simulink model "MicrogridControl"  (R2025b)
settings: Solver=VariableStepAuto  StartTime=0.0  StopTime=8  FixedStep=Ts  RelTol=1e-3
PreLoadFcn:
  | NormalOperation;
  | MicrogridControlParam;
undefined symbols (not defined in the file): base, bessModeInitial, bessSystem, bessVoltage, breakerStatus, DiscIntNeverNeededParam, ee_sli_rtmsupport, event, gcbh, generator, gflInverter, gfmInverter, Inertia, lineInductance, lineResistance, machine, plannedIsland, pmsm, powerLimit, powerQuality, PV, PVInverter, ref, resync, solar, solarInsolationChange, systemFrequency, Ts, windController, windSystem, windTurbine
libraries: nesl_utility x234, ee_lib x174, fl_lib x143, eeGeneralControl x137, simulink x78, eeTransforms x47, slpidlib x23, nesl_utility_internal x12, eePwmGenerator x9, eeSinusoidalMeasurementV2 x9, custom_lib x7, batteryecm_lib x6
(part 22 of 25)

== system MicrogridControl/Wind Farm/Wind Plant Integrated1/Detailed/Wind Turbine and Converters/Wind Plant/Back-to-Back Converters/Switching/Grid Side Converter ==
  mabc : Inport
  Add : Sum
  Constant1 : Constant
  Converter : ee_lib/Semiconductors & Converters/Converters/Converter (Three-Phase)  port_option=ee.enum.threePhasePort.composite  fidelity_option=ee.enum.converters.fidelity.detailed  device_type=ee.enum.converters.switchingdevice.ideal  showThermalPort=false  K=0  Vth=1 V  Vgt=1 V  Vgt_off=-1 V  Ih=1 A  Vf=0.8 V  Ron=0.001 Ohm  Rds=0.001 Ohm  Goff=1e-6 1/Ohm  Eon_scalar=22.86e-3 J  Eoff_scalar=17.14e-3 J  Eoff_natural_commutation=10e-3 J  Voff=300 V  Iout_scalar=600 A  onCurrentMeasDelay=0 s  useCurrentFromPreviousCycle=false  useVoltageFromPreviousCycle=false  diode_param=ee.enum.converters.protectiondiode.nodynamics  diode_Vf=0.01 V  diode_Ron=0.0001 Ohm  diode_Goff=1e-5 1/Ohm  diode_C=50 nF  diode_iRM=-235 A  diode_iF=300 A  diode_idot=-50 A/us  diode_trr_param=ee.enum.converters.diodetrr.trr_factor  diode_trr_factor=3  diode_trr=15 us  diode_Qrr=1500 s*uA  diode_rec_loss_model=ee.enum.diode.reverseRecoveryModel.fixed  diode_ErecVal=0 J  diode_scaleWithIandV=false  diode_ErecMat=zeros(2, 3) J  diode_TjrecVec=[298.15, 398.15] K  diode_IfrecVec=[.1, 1, 10] A  diode_IrecVal=10 A  diode_VrecVal=10 V  diode_tFilter=1 / 1000 / 100 s  thermal_network_parameterization=ee.enum.thermalNetworkTopology.external  Rth=[.08, .5] K/W  Rth_Cauer=[.08, .1, .5] K/W  Rth_Foster=[.08, .14, .22, .16] K/W  thermal_mass_parameterization=ee.enum.thermalNetwork.timeconstant  thermal_mass=[.01, .5] J/K  thermal_mass_Cauer=[.01, .1, .5] J/K  thermal_mass_Foster=[.001, .005, .05, .5] J/K  thermal_time_constant=[.001, .2] s  thermal_time_constant_Cauer=[.001, .1, .2] s  thermal_time_constant_Foster=[7e-05, .0007, .01, .08] s  thermal_mass_initial_temperatures=[25, 25] degC  thermal_mass_initial_temperatures_Cauer=[25, 25, 25] degC  junction_thermal_mass=0.01 J/K  Tvec_initial_Foster=[25, 25, 25, 25] degC  snubber_type=ee.enum.converters.snubber.exclude  Cs=1e-7 F  Rs=0.1 Ohm  Vce_loss=[0, 150, 300] V
  Demux : Demux  Outputs=3
  Demux1 : Demux  Outputs=3
  Gain : Gain  Gain=5
  Gain1 : Gain  Gain=0.5
  PWM Generator : eePwmGenerator/PWM Generator  CarrCount=Up  Tper=1/(fSw*1000)  Tdelay=0  Ts=1/(10*fSw*1000)
  Pulse Generation1 : Subsystem
  Rate Transition1 : RateTransition  OutPortSampleTime=1/(10*fSw*1000)
  Simulink-PS Converter{1..6} (6 alike) : nesl_utility/Simulink-PS Converter  PhysicalDomain=network_engine_domain  SubClassName=ps_input  LeftPortType=input  RightPortType=output  PseudoPeriodic=off  Frequencies=[]  NoiseDistribution=none  NoiseParameters=[]  Unit=1  AffineConversion=off  FilteringAndDerivatives=provide  SimscapeFilterOrder=1  InputFilterTimeConstant=0.001  UdotUserProvided=0
  Six-Pulse Gate Multiplexer : ee_lib/Semiconductors & Converters/Converters/Six-Pulse Gate Multiplexer  port_option=ee.enum.controlport.ps
  + : PMIOPort  Side=Left
  - : PMIOPort  Port=2  Side=Left
  ~ : PMIOPort  Port=3  Side=Right
  wires:
  [CH] -> Simulink-PS Converter2/1
  Demux/1 -> [AH]
  Add/1 -> Gain1/1
  Constant1/1 -> Add/2
  Demux/3 -> [CH]
  [AH] -> Simulink-PS Converter6/1
  Rate Transition1/1 -> PWM Generator/1
  [BH] -> Simulink-PS Converter4/1
  Demux1/3 -> [CL]
  [CL] -> Simulink-PS Converter1/1
  [AL] -> Simulink-PS Converter5/1
  PWM Generator/1 -> Gain/1
  Gain1/1 -> Rate Transition1/1
  Demux1/2 -> [BL]
  Demux/2 -> [BH]
  mabc/1 -> Add/1
  Gain/1 -> Pulse Generation1/1(G)
  Demux1/1 -> [AL]
  Pulse Generation1/2(G2) -> Demux1/1
  Pulse Generation1/1(G1) -> Demux/1
  [BL] -> Simulink-PS Converter3/1
  connections:
  +/RConn1 -- Converter/RConn1
  Six-Pulse Gate Multiplexer/LConn1 -- Simulink-PS Converter6/RConn1
  -/RConn1 -- Converter/RConn2
  Simulink-PS Converter2/RConn1 -- Six-Pulse Gate Multiplexer/LConn5
  Six-Pulse Gate Multiplexer/LConn3 -- Simulink-PS Converter4/RConn1
  Six-Pulse Gate Multiplexer/LConn2 -- Simulink-PS Converter5/RConn1
  Six-Pulse Gate Multiplexer/RConn1 -- Converter/LConn1
  ~/RConn1 -- Converter/LConn2
  Six-Pulse Gate Multiplexer/LConn4 -- Simulink-PS Converter3/RConn1
  Simulink-PS Converter1/RConn1 -- Six-Pulse Gate Multiplexer/LConn6

== system MicrogridControl/Wind Farm/Wind Plant Integrated1/Detailed/Wind Turbine and Converters/Wind Plant/Back-to-Back Converters/Switching/Machine Side Converter ==
  mabc : Inport
  Add : Sum
  Constant1 : Constant
  Converter : ee_lib/Semiconductors & Converters/Converters/Converter (Three-Phase)  port_option=ee.enum.threePhasePort.composite  fidelity_option=ee.enum.converters.fidelity.detailed  device_type=ee.enum.converters.switchingdevice.ideal  showThermalPort=false  K=0  Vth=1 V  Vgt=1 V  Vgt_off=-1 V  Ih=1 A  Vf=0.8 V  Ron=0.001 Ohm  Rds=0.001 Ohm  Goff=1e-6 1/Ohm  Eon_scalar=22.86e-3 J  Eoff_scalar=17.14e-3 J  Eoff_natural_commutation=10e-3 J  Voff=300 V  Iout_scalar=600 A  onCurrentMeasDelay=0 s  useCurrentFromPreviousCycle=false  useVoltageFromPreviousCycle=false  diode_param=ee.enum.converters.protectiondiode.nodynamics  diode_Vf=0.01 V  diode_Ron=0.0001 Ohm  diode_Goff=1e-5 1/Ohm  diode_C=50 nF  diode_iRM=-235 A  diode_iF=300 A  diode_idot=-50 A/us  diode_trr_param=ee.enum.converters.diodetrr.trr_factor  diode_trr_factor=3  diode_trr=15 us  diode_Qrr=1500 s*uA  diode_rec_loss_model=ee.enum.diode.reverseRecoveryModel.fixed  diode_ErecVal=0 J  diode_scaleWithIandV=false  diode_ErecMat=zeros(2, 3) J  diode_TjrecVec=[298.15, 398.15] K  diode_IfrecVec=[.1, 1, 10] A  diode_IrecVal=10 A  diode_VrecVal=10 V  diode_tFilter=1 / 1000 / 100 s  thermal_network_parameterization=ee.enum.thermalNetworkTopology.external  Rth=[.08, .5] K/W  Rth_Cauer=[.08, .1, .5] K/W  Rth_Foster=[.08, .14, .22, .16] K/W  thermal_mass_parameterization=ee.enum.thermalNetwork.timeconstant  thermal_mass=[.01, .5] J/K  thermal_mass_Cauer=[.01, .1, .5] J/K  thermal_mass_Foster=[.001, .005, .05, .5] J/K  thermal_time_constant=[.001, .2] s  thermal_time_constant_Cauer=[.001, .1, .2] s  thermal_time_constant_Foster=[7e-05, .0007, .01, .08] s  thermal_mass_initial_temperatures=[25, 25] degC  thermal_mass_initial_temperatures_Cauer=[25, 25, 25] degC  junction_thermal_mass=0.01 J/K  Tvec_initial_Foster=[25, 25, 25, 25] degC  snubber_type=ee.enum.converters.snubber.exclude  Cs=1e-7 F  Rs=0.1 Ohm  Vce_loss=[0, 150, 300] V
  Demux : Demux  Outputs=3
  Demux1 : Demux  Outputs=3
  Gain : Gain  Gain=5
  Gain1 : Gain  Gain=0.5
  PWM Generator : eePwmGenerator/PWM Generator  CarrCount=Up  Tper=1/(fSw*1000)  Tdelay=0  Ts=1/(10*fSw*1000)
  Pulse Generation : Subsystem
  Rate Transition1 : RateTransition  OutPortSampleTime=1/(10*fSw*1000)
  Simulink-PS Converter{1..6} (6 alike) : nesl_utility/Simulink-PS Converter  PhysicalDomain=network_engine_domain  SubClassName=ps_input  LeftPortType=input  RightPortType=output  PseudoPeriodic=off  Frequencies=[]  NoiseDistribution=none  NoiseParameters=[]  Unit=1  AffineConversion=off  FilteringAndDerivatives=provide  SimscapeFilterOrder=1  InputFilterTimeConstant=0.001  UdotUserProvided=0
  Six-Pulse Gate Multiplexer : ee_lib/Semiconductors & Converters/Converters/Six-Pulse Gate Multiplexer  port_option=ee.enum.controlport.ps
  + : PMIOPort  Side=Left
  - : PMIOPort  Port=2  Side=Left
  ~ : PMIOPort  Port=3  Side=Right
  wires:
  Demux1/1 -> [AL]
  Rate Transition1/1 -> PWM Generator/1
  Gain/1 -> Pulse Generation/1(G)
  [BH] -> Simulink-PS Converter4/1
  Gain1/1 -> Rate Transition1/1
  Demux/2 -> [BH]
  Pulse Generation/1(G1) -> Demux/1
  Pulse Generation/2(G2) -> Demux1/1
  PWM Generator/1 -> Gain/1
  Constant1/1 -> Add/2
  [AL] -> Simulink-PS Converter5/1
  Demux/3 -> [CH]
  [BL] -> Simulink-PS Converter3/1
  Demux/1 -> [AH]
  Add/1 -> Gain1/1
  Demux1/2 -> [BL]
  [CH] -> Simulink-PS Converter2/1
  Demux1/3 -> [CL]
  [CL] -> Simulink-PS Converter1/1
  mabc/1 -> Add/1
  [AH] -> Simulink-PS Converter6/1
  connections:
  Simulink-PS Converter2/RConn1 -- Six-Pulse Gate Multiplexer/LConn5
  ~/RConn1 -- Converter/LConn2
  Six-Pulse Gate Multiplexer/RConn1 -- Converter/LConn1
  Six-Pulse Gate Multiplexer/LConn2 -- Simulink-PS Converter5/RConn1
  Six-Pulse Gate Multiplexer/LConn4 -- Simulink-PS Converter3/RConn1
  -/RConn1 -- Converter/RConn2
  Six-Pulse Gate Multiplexer/LConn1 -- Simulink-PS Converter6/RConn1
  +/RConn1 -- Converter/RConn1
  Simulink-PS Converter1/RConn1 -- Six-Pulse Gate Multiplexer/LConn6
  Six-Pulse Gate Multiplexer/LConn3 -- Simulink-PS Converter4/RConn1

== system MicrogridControl/BESS/BESS Integrated/Detailed/BESS Controller/Grid Forming/Current Limiting/CurrentLimitingMethod/currentLimitAndVirtual/Current Saturation ==
  note: Vs-delV
  Id : Inport
  Iq : Inport  Port=2
  Imaxsat : Inport  Port=3
  Enable : EnablePort
  Compare : Subsystem
  Constant1 : Constant  Value=0
  Constant2 : Constant  Value=0
  If : If
  If Action Subsystem : Subsystem  TreatAsAtomicUnit=on
  If Action Subsystem1 : Subsystem  TreatAsAtomicUnit=on
  Math Function : Math  Operator=hypot
  Merge : Merge
  Merge1 : Merge
  Subtract : Sum  Inputs=+-
  delVd : Outport
  delVq : Outport  Port=2
  idmax : Outport  Port=3
  iqmax : Outport  Port=4
  wires:
  [Imax] -> If Action Subsystem/4(maxI)
  Imaxsat/1 -> Subtract/1, [Imax]
  Merge1/1 -> iqmax/1
  [Isq] -> If Action Subsystem/3(Isq)
  Constant1/1 -> delVd/1
  [Isd] -> If Action Subsystem/2(Isd)
  Merge/1 -> idmax/1
  If Action Subsystem1/2(Iqmax) -> Merge1/2
  Id/1 -> Math Function/1, [Isd]
  [Is] -> If Action Subsystem/1(Is)
  If Action Subsystem/1(Idmax) -> Merge/1
  Compare/1(Out1) -> If/1
  Subtract/1 -> Compare/1(u)
  If Action Subsystem/2(Iqmax) -> Merge1/1
  If/2 -> If Action Subsystem1/Action
  Math Function/1 -> Subtract/2, [Is]
  Constant2/1 -> delVq/1
  If Action Subsystem1/1(Idmax) -> Merge/2
  If/1 -> If Action Subsystem/Action
  Iq/1 -> Math Function/2, [Isq]

== system MicrogridControl/BESS/BESS Integrated/Detailed/BESS Controller/Grid Forming/Current Limiting/CurrentLimitingMethod/currentLimitAndVirtual/No Fault Ride Through ==
  Id : Inport
  Iq : Inport  Port=2
  Enable : EnablePort
  Constant{1..4} (4 alike) : Constant  Value=0
  Terminator : Terminator
  Terminator1 : Terminator
  delVd : Outport
  delVq : Outport  Port=2
  idmax : Outport  Port=3
  iqmax : Outport  Port=4
  wires:
  Iq/1 -> Terminator1/1
  Id/1 -> Terminator/1
  Constant4/1 -> delVq/1
  Constant1/1 -> delVd/1
  Constant2/1 -> idmax/1
  Constant3/1 -> iqmax/1

== system MicrogridControl/BESS/BESS Integrated/Detailed/BESS Controller/Grid Forming/Current Limiting/CurrentLimitingMethod/currentLimitAndVirtual/VI ==
  note: X/R ratio
  note: Resistance coefficient
  Id : Inport
  Iq : Inport  Port=2
  Imax : Inport  Port=3
  Enable : EnablePort
  Constant1 : Constant  Value=0
  Constant2 : Constant  Value=0
  Constant3 : Constant  Value=0
  Gain : Gain  Gain=ctLimitVirtualImp
  Gain1 : Gain  Gain=ctLimitXbyR
  Low-Pass Filter : eeGeneralControl/Low-Pass Filter (Discrete or Continuous)  K=1  T=currentVITimeConst  B=inf  A=-inf  init_option=Inherited from block input  x0=0  Ts=-1
  Math Function : Math  Operator=hypot
  Product{,1..3} (4 alike) : Product
  Relay1 : Relay  OnSwitchValue=0.01  OffSwitchValue=-0.1
  Saturation : Saturate  UpperLimit=1  LowerLimit=-1
  Saturation1 : Saturate  UpperLimit=1  LowerLimit=-1
  Sum : Sum  Inputs=|+-
  Sum1 : Sum  Inputs=|+-
  Sum2 : Sum  Inputs=++|
  Switch : Switch  Criteria=u2 > Threshold  SaturateOnIntegerOverflow=off  InputSameDT=off
  delVd : Outport
  delVq : Outport  Port=2
  idmax : Outport  Port=3
  iqmax : Outport  Port=4
  wires:
  Imax/1 -> Sum/2  "IsMaximum"
  Low-Pass Filter/1 -> Sum/1
  Relay1/1 -> Switch/2
  Constant2/1 -> idmax/1
  Constant3/1 -> iqmax/1
  Saturation/1 -> delVd/1
  Constant1/1 -> Switch/3
  Gain/1 -> Switch/1
  Product2/1 -> Sum1/2
  Product1/1 -> Sum2/1
  Saturation1/1 -> delVq/1
  [Igd] -> Product/2, Product1/1
  Switch/1 -> Gain1/1, Product/1, Product3/2
  Math Function/1 -> Low-Pass Filter/1  "Is"
  Iq/1 -> Math Function/2, [Igq]
  [Igq] -> Product2/2, Product3/1
  Product/1 -> Sum1/1
  Sum1/1 -> Saturation/1
  Sum/1 -> Relay1/1, Gain/1
  Sum2/1 -> Saturation1/1
  Id/1 -> [Igd], Math Function/1
  Product3/1 -> Sum2/2
  Gain1/1 -> Product2/1, Product1/2

== system MicrogridControl/BESS/BESS Integrated/Detailed/BESS Controller/Grid Forming/Current Limiting/CurrentLimitingMethod/currentSaturation/Compare ==
  u : Inport
  AND : Logic  IconShape=distinctive  AllPortsSameDT=off  OutDataTypeStr=boolean
  Compare To Constant : simulink/Logic and Bit Operations/Compare To Constant  relop=>  const=ctLimitDelayTime  OutDataTypeStr=boolean
  Compare To Zero : simulink/Logic and Bit Operations/Compare To Zero  relop=<=  OutDataTypeStr=boolean
  Data Type Conversion : DataTypeConversion  SaturateOnIntegerOverflow=off  RndMeth=Floor
  Data Type Conversion1 : DataTypeConversion  SaturateOnIntegerOverflow=off  RndMeth=Floor
  Discrete-Time Integrator : DiscreteIntegrator  IntegratorMethod=Integration: Backward Euler  ExternalReset=level  SampleTime=currentControlTs  LimitOutput=on  UpperSaturationLimit=ctLimitDelayTime*2  LowerSaturationLimit=0  ICPrevOutput=DiscIntNeverNeededParam  ICPrevScaledInput=DiscIntNeverNeededParam
  Out1 : Outport
  wires:
  Data Type Conversion1/1 -> AND/1, Discrete-Time Integrator/1, Discrete-Time Integrator/2
  Data Type Conversion/1 -> Out1/1
  Discrete-Time Integrator/1 -> Compare To Constant/1
  u/1 -> Compare To Zero/1
  Compare To Constant/1 -> AND/2
  Compare To Zero/1 -> Data Type Conversion1/1
  AND/1 -> Data Type Conversion/1

== system MicrogridControl/BESS/BESS Integrated/Detailed/BESS Controller/Grid Forming/Current Limiting/CurrentLimitingMethod/currentSaturation/If Action Subsystem ==
  Is : Inport
  Isd : Inport  Port=2
  Isq : Inport  Port=3
  Action Port : ActionPort  ActionPortLabel=if(u1 > 0)
  Constant : Constant  Value=maxSatCurrentLimit
  Divide : Product  Inputs=*/
  Product : Product
  Product1 : Product
  Idmax : Outport
  Iqmax : Outport  Port=2
  wires:
  Product/1 -> Iqmax/1
  Product1/1 -> Idmax/1
  Isq/1 -> Product/2
  Isd/1 -> Product1/1
  Divide/1 -> Product/1, Product1/2
  Is/1 -> Divide/2
  Constant/1 -> Divide/1

== system MicrogridControl/BESS/BESS Integrated/Detailed/BESS Controller/Grid Forming/Current Limiting/CurrentLimitingMethod/currentSaturation/If Action Subsystem1 ==
  Action Port : ActionPort  ActionPortLabel=else
  Constant3 : Constant  Value=0
  Constant4 : Constant  Value=0
  Idmax : Outport
  Iqmax : Outport  Port=2
  wires:
  Constant3/1 -> Idmax/1
  Constant4/1 -> Iqmax/1

== system MicrogridControl/BESS/BESS Integrated/Detailed/BESS Controller/Grid Forming/Grid Voltage Reactive Power Support/Modifying Reactive Power Reference/Changing the Power Reference/ActivePowerReference ==
  note: Ensure Pref sign is maintained
  Id : Inport
  Vd : Inport  Port=2
  Pref : Inport  Port=3
  Abs1 : Abs  SaturateOnIntegerOverflow=off
  Abs2 : Abs  SaturateOnIntegerOverflow=off
  Min : MinMax  Inputs=2
  Product : Product
  Product2 : Product
  Saturation : Saturate  UpperLimit=1  LowerLimit=-1
  Sign : Signum
  PrefNew : Outport
  wires:
  Saturation/1 -> PrefNew/1
  Vd/1 -> Product/2
  Abs2/1 -> Min/1
  Product2/1 -> Saturation/1
  Min/1 -> Product2/1
  Product/1 -> Abs2/1
  Abs1/1 -> Min/2
  Sign/1 -> Product2/2
  Id/1 -> Product/1
  Pref/1 -> Sign/1, Abs1/1

== system MicrogridControl/BESS/BESS Integrated/Detailed/BESS Controller/Grid Forming/Grid Voltage Reactive Power Support/Modifying Reactive Power Reference/Changing the Power Reference/EstimateIdForGivenIq ==
  Iq : Inport
  Add Constant1 : Bias  Bias=1*1  SaturateOnIntegerOverflow=off
  Gain : Gain  Gain=-1
  Gain3 : Gain  Gain=0.9
  Sqrt : Sqrt
  Square : Math  Operator=square
  Id : Outport
  wires:
  Iq/1 -> Square/1
  Add Constant1/1 -> Sqrt/1
  Sqrt/1 -> Gain3/1
  Gain/1 -> Add Constant1/1
  Gain3/1 -> Id/1
  Square/1 -> Gain/1

== system MicrogridControl/BESS/BESS Integrated/Detailed/BESS Controller/Grid Forming/Grid Voltage Reactive Power Support/Modifying Reactive Power Reference/Changing the Power Reference/EstimateIqForReactivePower ==
  note: Computing minimum reactive power as per GC0137
  Vmin : Inport
  Vd : Inport  Port=2
  Vs : Inport  Port=3
  Abs : Abs  SaturateOnIntegerOverflow=off
  Add : Sum
  Add Constant : Bias  Bias=1  SaturateOnIntegerOverflow=off
  GC0137 line slope : Gain  Gain=-1.4578
  Gain4 : Gain  Gain=1.5
  Saturation : Saturate  UpperLimit=1  LowerLimit=0
  Saturation1 : Saturate  UpperLimit=1  LowerLimit=-1
  Subtract : Sum  Inputs=+-
  Iq : Outport
  wires:
  Add Constant/1 -> Add/2
  Saturation/1 -> Iq/1
  Add/1 -> Saturation/1
  Vd/1 -> Subtract/2
  Vs/1 -> Abs/1
  Vmin/1 -> Subtract/1
  Gain4/1 -> Saturation1/1
  Saturation1/1 -> Add/1
  Subtract/1 -> Gain4/1
  GC0137 line slope/1 -> Add Constant/1
  Abs/1 -> GC0137 line slope/1

== system MicrogridControl/BESS/BESS Integrated/Detailed/BESS Controller/Grid Forming/Grid Voltage Reactive Power Support/Modifying Reactive Power Reference/Changing the Power Reference/ReactivePowerReference ==
  Vd : Inport
  Iq : Inport  Port=2
  Compute Power : Product
  Constant : Constant  Value=0.3
  Gain2 : Gain  Gain=1.05
  Switch : Switch  Criteria=u2 > Threshold  Threshold=0.3  SaturateOnIntegerOverflow=off  InputSameDT=off
  QrefNew : Outport
  wires:
  Switch/1 -> Compute Power/1
  Vd/1 -> Switch/1, Switch/2
  Iq/1 -> Gain2/1
  Constant/1 -> Switch/3
  Gain2/1 -> Compute Power/2
  Compute Power/1 -> QrefNew/1

== system MicrogridControl/BESS/BESS Integrated/Detailed/BESS Controller/Grid Forming/Measurement/Frequency Measurement/Frequency Measurement/If Action Subsystem ==
  V : Inport
  Time : Inport  Port=2
  Action Port : ActionPort  ActionPortLabel=if(u1 > 0.9)
  Constant1 : Constant  Value=initialFrequency
  Delay : Delay  DelayLength=1
  Delay1 : Delay  DelayLength=1
  Frequency estimation : Subsystem  TreatAsAtomicUnit=on
  Hit Crossing : HitCross
  Second-Order Filter : eeGeneralControl/Second-Order Filter  Commented=through  FilterType=Low-pass  fn=initialFrequency  Zeta=1  Ts=sampleTime  A0=0  Ph0=0  f0=0  b0=0
  Switch : Switch  Criteria=u2 > Threshold  Threshold=1  SaturateOnIntegerOverflow=off  InputSameDT=off
  Freq : Outport
  wires:
  Switch/1 -> Freq/1
  Constant1/1 -> Switch/3
  Frequency estimation/1(f) -> Switch/1
  Time/1 -> Frequency estimation/3(k), Delay1/1, Switch/2
  V/1 -> Second-Order Filter/1
  Delay/1 -> Frequency estimation/2(sk-1)
  Hit Crossing/1 -> Frequency estimation/Trigger
  Delay1/1 -> Frequency estimation/4(k-1)
  Second-Order Filter/1 -> Hit Crossing/1, Frequency estimation/1(sk), Delay/1

== system MicrogridControl/BESS/BESS Integrated/Detailed/BESS Controller/Grid Forming/Measurement/Frequency Measurement/Frequency Measurement/If Action Subsystem1 ==
  Action Port : ActionPort  ActionPortLabel=else
  Constant1 : Constant  Value=initialFrequency
  Out1 : Outport
  wires:
  Constant1/1 -> Out1/1

== system MicrogridControl/BESS/BESS Integrated/Detailed/BESS Controller/Grid Forming/Measurement/Frequency Measurement/Frequency Measurement/Postive Sequence ==
  abc : Inport
  Complex to Real-Imag : ComplexToRealImag
  Demux : Demux  Outputs=3
  Symmetrical-Components Transform : eeTransforms/Symmetrical-Components Transform  PowerInvariant=off
  Terminator : Terminator
  Terminator1 : Terminator
  Terminator2 : Terminator
  Transpose : Math  Operator=transpose
  posSeq : Outport
  wires:
  Demux/3 -> Terminator2/1
  Demux/2 -> Terminator1/1
  Complex to Real-Imag/2 -> Terminator/1
  abc/1 -> Transpose/1
  Demux/1 -> Complex to Real-Imag/1
  Complex to Real-Imag/1 -> posSeq/1
  Symmetrical-Components Transform/1 -> Demux/1
  Transpose/1 -> Symmetrical-Components Transform/1

== system MicrogridControl/BESS/BESS Integrated/Detailed/BESS Controller/Grid Forming/Power Control/ActivePowerControl/vsmControl/Damping Frequency ==
  fref : Inport
  ConstantFreqReference : Subsystem  VariantControl=constFreq
  WithFrequencyMeasurement : Subsystem  VariantControl=freqMeas
  fmeas : Outport

== system MicrogridControl/BESS/BESS Integrated/Detailed/BESS Controller/Grid Forming/Power Control/ActivePowerControl/vsmControl/Power Reference Selection ==
  cntrlflag : Inport
  Pref : Inport  Port=2
  fref : Inport  Port=3
  Wsm : Inport  Port=4
  If : If
  If Action Subsystem : Subsystem  TreatAsAtomicUnit=on
  If Action Subsystem1 : Subsystem  TreatAsAtomicUnit=on
  Merge : Merge
  Scope : Scope
      settings: ActiveDisplayYMinimum=-1  ActiveDisplayYMaximum=1
  power : Outport
  wires:
  Wsm/1 -> [Wsm]
  Merge/1 -> power/1, Scope/1
  cntrlflag/1 -> If/1
  If/2 -> If Action Subsystem1/Action
  If Action Subsystem/1(Power) -> Merge/1
  [Wsm] -> If Action Subsystem/2(Wsm)
  fref/1 -> If Action Subsystem1/1(fref)
  [Wsm] -> If Action Subsystem1/2(Wsm)
  Pref/1 -> If Action Subsystem/1(Pref)
  If/1 -> If Action Subsystem/Action
  If Action Subsystem1/1(Power) -> Merge/2

== system MicrogridControl/BESS/BESS Integrated/Detailed/BESS Controller/Grid Forming/Power Control/ReactiveControl/Voltage  Reference Selection/If Action Subsystem ==
  note: Vs-delV
  Qref : Inport
  Qmeas : Inport  Port=2
  Action Port : ActionPort  ActionPortLabel=if(u1 > 0)
  Constant : Constant  Value=voltreference
  Gain : Gain  Gain=QVoltDroop
  Low-Pass Filter (Discrete or Continuous) : eeGeneralControl/Low-Pass Filter (Discrete or Continuous)  K=1  T=QVoltFilterTC  B=inf  A=-inf  init_option=Specify as parameter  x0=0  Ts=activePowerSampleTime
  Product1 : Product
  Scope : Scope
      settings: ActiveDisplayYMinimum=-1  ActiveDisplayYMaximum=1
  Scope1 : Scope  NumInputPorts=2
      settings: ActiveDisplayYMinimum=-0.71158  ActiveDisplayYMaximum=0.42604  DataLoggingVariableName=ScopeData5
  Sum : Sum  Inputs=|+-
  Sum1 : Sum  Inputs=|++
  Vd : Outport
  wires:
  Product1/1 -> Vd/1  "V"
  Sum1/1 -> Product1/1
  Sum/1 -> Gain/1
  Low-Pass Filter (Discrete or Continuous)/1 -> Sum/2
  Qref/1 -> Scope1/1, Sum/1
  Gain/1 -> Sum1/1, Scope/1
  Qmeas/1 -> Scope1/2, Low-Pass Filter (Discrete or Continuous)/1
  Constant/1 -> Sum1/2, Product1/2

== system MicrogridControl/BESS/BESS Integrated/Detailed/BESS Controller/Grid Forming/Power Control/ReactiveControl/Voltage  Reference Selection/If Action Subsystem1 ==
  note: Vs-delV
  Vref : Inport
  Vmeas : Inport  Port=2
  Action Port : ActionPort  ActionPortLabel=else
  Constant : Constant  Value=voltreference
  Gain : Gain  Gain=1e-3/QVoltDroop
  Low-Pass Filter (Discrete or Continuous) : eeGeneralControl/Low-Pass Filter (Discrete or Continuous)  K=1  T=QVoltFilterTC  B=inf  A=-inf  init_option=Specify as parameter  x0=0  Ts=activePowerSampleTime
  Product1 : Product
  Scope : Scope
      settings: ActiveDisplayYMinimum=8.18716  ActiveDisplayYMaximum=11.15581  DataLoggingVariableName=ScopeData11  DataLoggingSaveFormat=Array
  Scope1 : Scope
      settings: ActiveDisplayYMinimum=0.78014  ActiveDisplayYMaximum=0.78049  DataLoggingVariableName=ScopeData12  DataLoggingSaveFormat=Array
  Scope2 : Scope  NumInputPorts=2
      settings: ActiveDisplayYMinimum=0.83186  ActiveDisplayYMaximum=1.08242  DataLoggingVariableName=ScopeData13  DataLoggingSaveFormat=Array
  Sum : Sum  Inputs=|+-
  Sum1 : Sum  Inputs=|++
  Voltage : Outport
  wires:
  Sum1/1 -> Product1/2
  Product1/1 -> Scope/1, Voltage/1  "V"
  Sum/1 -> Gain/1
  Low-Pass Filter (Discrete or Continuous)/1 -> Scope1/1, Sum/2
  Constant/1 -> Sum1/2
  Vmeas/1 -> Low-Pass Filter (Discrete or Continuous)/1, Scope2/2
  Gain/1 -> Sum1/1
  Vref/1 -> Sum/1, Product1/1, Scope2/1

== system MicrogridControl/BESS/BESS Integrated1/Detailed/BESS Controller/Grid Forming/Current Limiting/CurrentLimitingMethod/currentLimitAndVirtual/Current Saturation ==
  note: Vs-delV
  Id : Inport
  Iq : Inport  Port=2
  Imaxsat : Inport  Port=3
  Enable : EnablePort
  Compare : Subsystem
  Constant1 : Constant  Value=0
  Constant2 : Constant  Value=0
  If : If
  If Action Subsystem : Subsystem  TreatAsAtomicUnit=on
  If Action Subsystem1 : Subsystem  TreatAsAtomicUnit=on
  Math Function : Math  Operator=hypot
  Merge : Merge
  Merge1 : Merge
  Subtract : Sum  Inputs=+-
  delVd : Outport
  delVq : Outport  Port=2
  idmax : Outport  Port=3
  iqmax : Outport  Port=4
  wires:
  [Imax] -> If Action Subsystem/4(maxI)
  Imaxsat/1 -> Subtract/1, [Imax]
  Merge1/1 -> iqmax/1
  [Isq] -> If Action Subsystem/3(Isq)
  Constant1/1 -> delVd/1
  [Isd] -> If Action Subsystem/2(Isd)
  Merge/1 -> idmax/1
  If Action Subsystem1/2(Iqmax) -> Merge1/2
  Id/1 -> Math Function/1, [Isd]
  [Is] -> If Action Subsystem/1(Is)
  If Action Subsystem/1(Idmax) -> Merge/1
  Compare/1(Out1) -> If/1
  Subtract/1 -> Compare/1(u)
  If Action Subsystem/2(Iqmax) -> Merge1/1
  If/2 -> If Action Subsystem1/Action
  Math Function/1 -> Subtract/2, [Is]
  Constant2/1 -> delVq/1
  If Action Subsystem1/1(Idmax) -> Merge/2
  If/1 -> If Action Subsystem/Action
  Iq/1 -> Math Function/2, [Isq]

== system MicrogridControl/BESS/BESS Integrated1/Detailed/BESS Controller/Grid Forming/Current Limiting/CurrentLimitingMethod/currentLimitAndVirtual/No Fault Ride Through ==
  Id : Inport
  Iq : Inport  Port=2
  Enable : EnablePort
  Constant{1..4} (4 alike) : Constant  Value=0
  Terminator : Terminator
  Terminator1 : Terminator
  delVd : Outport
  delVq : Outport  Port=2
  idmax : Outport  Port=3
  iqmax : Outport  Port=4
  wires:
  Iq/1 -> Terminator1/1
  Id/1 -> Terminator/1
  Constant4/1 -> delVq/1
  Constant1/1 -> delVd/1
  Constant2/1 -> idmax/1
  Constant3/1 -> iqmax/1

== system MicrogridControl/BESS/BESS Integrated1/Detailed/BESS Controller/Grid Forming/Current Limiting/CurrentLimitingMethod/currentLimitAndVirtual/VI ==
  note: X/R ratio
  note: Resistance coefficient
  Id : Inport
  Iq : Inport  Port=2
  Imax : Inport  Port=3
  Enable : EnablePort
  Constant1 : Constant  Value=0
  Constant2 : Constant  Value=0
  Constant3 : Constant  Value=0
  Gain : Gain  Gain=ctLimitVirtualImp
  Gain1 : Gain  Gain=ctLimitXbyR
  Low-Pass Filter : eeGeneralControl/Low-Pass Filter (Discrete or Continuous)  K=1  T=currentVITimeConst  B=inf  A=-inf  init_option=Inherited from block input  x0=0  Ts=-1
  Math Function : Math  Operator=hypot
  Product{,1..3} (4 alike) : Product
  Relay1 : Relay  OnSwitchValue=0.01  OffSwitchValue=-0.1
  Saturation : Saturate  UpperLimit=1  LowerLimit=-1
  Saturation1 : Saturate  UpperLimit=1  LowerLimit=-1
  Sum : Sum  Inputs=|+-
  Sum1 : Sum  Inputs=|+-
  Sum2 : Sum  Inputs=++|
  Switch : Switch  Criteria=u2 > Threshold  SaturateOnIntegerOverflow=off  InputSameDT=off
  delVd : Outport
  delVq : Outport  Port=2
  idmax : Outport  Port=3
  iqmax : Outport  Port=4
  wires:
  Imax/1 -> Sum/2  "IsMaximum"
  Low-Pass Filter/1 -> Sum/1
  Relay1/1 -> Switch/2
  Constant2/1 -> idmax/1
  Constant3/1 -> iqmax/1
  Saturation/1 -> delVd/1
  Constant1/1 -> Switch/3
  Gain/1 -> Switch/1
  Product2/1 -> Sum1/2
  Product1/1 -> Sum2/1
  Saturation1/1 -> delVq/1
  [Igd] -> Product/2, Product1/1
  Switch/1 -> Gain1/1, Product/1, Product3/2
  Math Function/1 -> Low-Pass Filter/1  "Is"
  Iq/1 -> Math Function/2, [Igq]
  [Igq] -> Product2/2, Product3/1
  Product/1 -> Sum1/1
  Sum1/1 -> Saturation/1
  Sum/1 -> Relay1/1, Gain/1
  Sum2/1 -> Saturation1/1
  Id/1 -> [Igd], Math Function/1
  Product3/1 -> Sum2/2
  Gain1/1 -> Product2/1, Product1/2

== system MicrogridControl/BESS/BESS Integrated1/Detailed/BESS Controller/Grid Forming/Current Limiting/CurrentLimitingMethod/currentSaturation/Compare ==
  u : Inport
  AND : Logic  IconShape=distinctive  AllPortsSameDT=off  OutDataTypeStr=boolean
  Compare To Constant : simulink/Logic and Bit Operations/Compare To Constant  relop=>  const=ctLimitDelayTime  OutDataTypeStr=boolean
  Compare To Zero : simulink/Logic and Bit Operations/Compare To Zero  relop=<=  OutDataTypeStr=boolean
  Data Type Conversion : DataTypeConversion  SaturateOnIntegerOverflow=off  RndMeth=Floor
  Data Type Conversion1 : DataTypeConversion  SaturateOnIntegerOverflow=off  RndMeth=Floor
  Discrete-Time Integrator : DiscreteIntegrator  IntegratorMethod=Integration: Backward Euler  ExternalReset=level  SampleTime=currentControlTs  LimitOutput=on  UpperSaturationLimit=ctLimitDelayTime*2  LowerSaturationLimit=0  ICPrevOutput=DiscIntNeverNeededParam  ICPrevScaledInput=DiscIntNeverNeededParam
  Out1 : Outport
  wires:
  Data Type Conversion1/1 -> AND/1, Discrete-Time Integrator/1, Discrete-Time Integrator/2
  Data Type Conversion/1 -> Out1/1
  Discrete-Time Integrator/1 -> Compare To Constant/1
  u/1 -> Compare To Zero/1
  Compare To Constant/1 -> AND/2
  Compare To Zero/1 -> Data Type Conversion1/1
  AND/1 -> Data Type Conversion/1

== system MicrogridControl/BESS/BESS Integrated1/Detailed/BESS Controller/Grid Forming/Current Limiting/CurrentLimitingMethod/currentSaturation/If Action Subsystem ==
  Is : Inport
  Isd : Inport  Port=2
  Isq : Inport  Port=3
  Action Port : ActionPort  ActionPortLabel=if(u1 > 0)
  Constant : Constant  Value=maxSatCurrentLimit
  Divide : Product  Inputs=*/
  Product : Product
  Product1 : Product
  Idmax : Outport
  Iqmax : Outport  Port=2
  wires:
  Product/1 -> Iqmax/1
  Product1/1 -> Idmax/1
  Isq/1 -> Product/2
  Isd/1 -> Product1/1
  Divide/1 -> Product/1, Product1/2
  Is/1 -> Divide/2
  Constant/1 -> Divide/1

== system MicrogridControl/BESS/BESS Integrated1/Detailed/BESS Controller/Grid Forming/Current Limiting/CurrentLimitingMethod/currentSaturation/If Action Subsystem1 ==
  Action Port : ActionPort  ActionPortLabel=else
  Constant3 : Constant  Value=0
  Constant4 : Constant  Value=0
  Idmax : Outport
  Iqmax : Outport  Port=2
  wires:
  Constant3/1 -> Idmax/1
  Constant4/1 -> Iqmax/1

== system MicrogridControl/BESS/BESS Integrated1/Detailed/BESS Controller/Grid Forming/Grid Voltage Reactive Power Support/Modifying Reactive Power Reference/Changing the Power Reference/ActivePowerReference ==
  note: Ensure Pref sign is maintained
  Id : Inport
  Vd : Inport  Port=2
  Pref : Inport  Port=3
  Abs1 : Abs  SaturateOnIntegerOverflow=off
  Abs2 : Abs  SaturateOnIntegerOverflow=off
  Min : MinMax  Inputs=2
  Product : Product
  Product2 : Product
  Saturation : Saturate  UpperLimit=1  LowerLimit=-1
  Sign : Signum
  PrefNew : Outport
  wires:
  Saturation/1 -> PrefNew/1
  Vd/1 -> Product/2
  Abs2/1 -> Min/1
  Product2/1 -> Saturation/1
  Min/1 -> Product2/1
  Product/1 -> Abs2/1
  Abs1/1 -> Min/2
  Sign/1 -> Product2/2
  Id/1 -> Product/1
  Pref/1 -> Sign/1, Abs1/1

== system MicrogridControl/BESS/BESS Integrated1/Detailed/BESS Controller/Grid Forming/Grid Voltage Reactive Power Support/Modifying Reactive Power Reference/Changing the Power Reference/EstimateIdForGivenIq ==
  Iq : Inport
  Add Constant1 : Bias  Bias=1*1  SaturateOnIntegerOverflow=off
  Gain : Gain  Gain=-1
  Gain3 : Gain  Gain=0.9
  Sqrt : Sqrt
  Square : Math  Operator=square
  Id : Outport
  wires:
  Iq/1 -> Square/1
  Add Constant1/1 -> Sqrt/1
  Sqrt/1 -> Gain3/1
  Gain/1 -> Add Constant1/1
  Gain3/1 -> Id/1
  Square/1 -> Gain/1

== system MicrogridControl/BESS/BESS Integrated1/Detailed/BESS Controller/Grid Forming/Grid Voltage Reactive Power Support/Modifying Reactive Power Reference/Changing the Power Reference/EstimateIqForReactivePower ==
  note: Computing minimum reactive power as per GC0137
  Vmin : Inport
  Vd : Inport  Port=2
  Vs : Inport  Port=3
  Abs : Abs  SaturateOnIntegerOverflow=off
  Add : Sum
  Add Constant : Bias  Bias=1  SaturateOnIntegerOverflow=off
  GC0137 line slope : Gain  Gain=-1.4578
  Gain4 : Gain  Gain=1.5
  Saturation : Saturate  UpperLimit=1  LowerLimit=0
  Saturation1 : Saturate  UpperLimit=1  LowerLimit=-1
  Subtract : Sum  Inputs=+-
  Iq : Outport
  wires:
  Add Constant/1 -> Add/2
  Saturation/1 -> Iq/1
  Add/1 -> Saturation/1
  Vd/1 -> Subtract/2
  Vs/1 -> Abs/1
  Vmin/1 -> Subtract/1
  Gain4/1 -> Saturation1/1
  Saturation1/1 -> Add/1
  Subtract/1 -> Gain4/1
  GC0137 line slope/1 -> Add Constant/1
  Abs/1 -> GC0137 line slope/1

== system MicrogridControl/BESS/BESS Integrated1/Detailed/BESS Controller/Grid Forming/Grid Voltage Reactive Power Support/Modifying Reactive Power Reference/Changing the Power Reference/ReactivePowerReference ==
  Vd : Inport
  Iq : Inport  Port=2
  Compute Power : Product
  Constant : Constant  Value=0.3
  Gain2 : Gain  Gain=1.05
  Switch : Switch  Criteria=u2 > Threshold  Threshold=0.3  SaturateOnIntegerOverflow=off  InputSameDT=off
  QrefNew : Outport
  wires:
  Switch/1 -> Compute Power/1
  Vd/1 -> Switch/1, Switch/2
  Iq/1 -> Gain2/1
  Constant/1 -> Switch/3
  Gain2/1 -> Compute Power/2
  Compute Power/1 -> QrefNew/1

== system MicrogridControl/BESS/BESS Integrated1/Detailed/BESS Controller/Grid Forming/Measurement/Frequency Measurement/Frequency Measurement/If Action Subsystem ==
  V : Inport
  Time : Inport  Port=2
  Action Port : ActionPort  ActionPortLabel=if(u1 > 0.9)
  Constant1 : Constant  Value=initialFrequency
  Delay : Delay  DelayLength=1
  Delay1 : Delay  DelayLength=1
  Frequency estimation : Subsystem  TreatAsAtomicUnit=on
  Hit Crossing : HitCross
  Second-Order Filter : eeGeneralControl/Second-Order Filter  Commented=through  FilterType=Low-pass  fn=initialFrequency  Zeta=1  Ts=sampleTime  A0=0  Ph0=0  f0=0  b0=0
  Switch : Switch  Criteria=u2 > Threshold  Threshold=1  SaturateOnIntegerOverflow=off  InputSameDT=off
  Freq : Outport
  wires:
  Switch/1 -> Freq/1
  Constant1/1 -> Switch/3
  Frequency estimation/1(f) -> Switch/1
  Time/1 -> Frequency estimation/3(k), Delay1/1, Switch/2
  V/1 -> Second-Order Filter/1
  Delay/1 -> Frequency estimation/2(sk-1)
  Hit Crossing/1 -> Frequency estimation/Trigger
  Delay1/1 -> Frequency estimation/4(k-1)
  Second-Order Filter/1 -> Hit Crossing/1, Frequency estimation/1(sk), Delay/1

== system MicrogridControl/BESS/BESS Integrated1/Detailed/BESS Controller/Grid Forming/Measurement/Frequency Measurement/Frequency Measurement/If Action Subsystem1 ==
  Action Port : ActionPort  ActionPortLabel=else
  Constant1 : Constant  Value=initialFrequency
  Out1 : Outport
  wires:
  Constant1/1 -> Out1/1

== system MicrogridControl/BESS/BESS Integrated1/Detailed/BESS Controller/Grid Forming/Measurement/Frequency Measurement/Frequency Measurement/Postive Sequence ==
  abc : Inport
  Complex to Real-Imag : ComplexToRealImag
  Demux : Demux  Outputs=3
  Symmetrical-Components Transform : eeTransforms/Symmetrical-Components Transform  PowerInvariant=off
  Terminator : Terminator
  Terminator1 : Terminator
  Terminator2 : Terminator
  Transpose : Math  Operator=transpose
  posSeq : Outport
  wires:
  Demux/3 -> Terminator2/1
  Demux/2 -> Terminator1/1
  Complex to Real-Imag/2 -> Terminator/1
  abc/1 -> Transpose/1
  Demux/1 -> Complex to Real-Imag/1
  Complex to Real-Imag/1 -> posSeq/1
  Symmetrical-Components Transform/1 -> Demux/1
  Transpose/1 -> Symmetrical-Components Transform/1

== system MicrogridControl/BESS/BESS Integrated1/Detailed/BESS Controller/Grid Forming/Power Control/ActivePowerControl/vsmControl/Damping Frequency ==
  fref : Inport
  ConstantFreqReference : Subsystem  VariantControl=constFreq
  WithFrequencyMeasurement : Subsystem  VariantControl=freqMeas
  fmeas : Outport

== system MicrogridControl/BESS/BESS Integrated1/Detailed/BESS Controller/Grid Forming/Power Control/ActivePowerControl/vsmControl/Power Reference Selection ==
  cntrlflag : Inport
  Pref : Inport  Port=2
  fref : Inport  Port=3
  Wsm : Inport  Port=4
  If : If
  If Action Subsystem : Subsystem  TreatAsAtomicUnit=on
  If Action Subsystem1 : Subsystem  TreatAsAtomicUnit=on
  Merge : Merge
  Scope : Scope
  power : Outport
  wires:
  Wsm/1 -> [Wsm]
  Merge/1 -> power/1, Scope/1
  cntrlflag/1 -> If/1
  If/2 -> If Action Subsystem1/Action
  If Action Subsystem/1(Power) -> Merge/1
  [Wsm] -> If Action Subsystem/2(Wsm)
  fref/1 -> If Action Subsystem1/1(fref)
  [Wsm] -> If Action Subsystem1/2(Wsm)
  Pref/1 -> If Action Subsystem/1(Pref)
  If/1 -> If Action Subsystem/Action
  If Action Subsystem1/1(Power) -> Merge/2

== system MicrogridControl/BESS/BESS Integrated1/Detailed/BESS Controller/Grid Forming/Power Control/ReactiveControl/Voltage  Reference Selection/If Action Subsystem ==
  note: Vs-delV
  Qref : Inport
  Qmeas : Inport  Port=2
  Action Port : ActionPort  ActionPortLabel=if(u1 > 0)
  Constant : Constant  Value=voltreference
  Gain : Gain  Gain=QVoltDroop
  Low-Pass Filter (Discrete or Continuous) : eeGeneralControl/Low-Pass Filter (Discrete or Continuous)  K=1  T=QVoltFilterTC  B=inf  A=-inf  init_option=Specify as parameter  x0=0  Ts=activePowerSampleTime
  Product1 : Product
  Scope : Scope
      settings: ActiveDisplayYMinimum=-0.00042  ActiveDisplayYMaximum=0.0007
  Scope1 : Scope  NumInputPorts=2
      settings: ActiveDisplayYMinimum=-0.71158  ActiveDisplayYMaximum=0.42604  DataLoggingVariableName=ScopeData5
  Sum : Sum  Inputs=|+-
  Sum1 : Sum  Inputs=|++
  Vd : Outport
  wires:
  Product1/1 -> Vd/1  "V"
  Sum1/1 -> Product1/1
  Sum/1 -> Gain/1
  Low-Pass Filter (Discrete or Continuous)/1 -> Sum/2
  Qref/1 -> Scope1/1, Sum/1
  Gain/1 -> Sum1/1, Scope/1
  Qmeas/1 -> Scope1/2, Low-Pass Filter (Discrete or Continuous)/1
  Constant/1 -> Sum1/2, Product1/2

== system MicrogridControl/BESS/BESS Integrated1/Detailed/BESS Controller/Grid Forming/Power Control/ReactiveControl/Voltage  Reference Selection/If Action Subsystem1 ==
  note: Vs-delV
  Vref : Inport
  Vmeas : Inport  Port=2
  Action Port : ActionPort  ActionPortLabel=else
  Constant : Constant  Value=voltreference
  Gain : Gain  Gain=1e-3/QVoltDroop
  Low-Pass Filter (Discrete or Continuous) : eeGeneralControl/Low-Pass Filter (Discrete or Continuous)  K=1  T=QVoltFilterTC  B=inf  A=-inf  init_option=Specify as parameter  x0=0  Ts=activePowerSampleTime
  Product1 : Product
  Scope : Scope
      settings: ActiveDisplayYMinimum=8.18716  ActiveDisplayYMaximum=11.15581  DataLoggingVariableName=ScopeData11  DataLoggingSaveFormat=Array
  Scope1 : Scope
      settings: ActiveDisplayYMinimum=0.78014  ActiveDisplayYMaximum=0.78049  DataLoggingVariableName=ScopeData12  DataLoggingSaveFormat=Array
  Scope2 : Scope  NumInputPorts=2
      settings: ActiveDisplayYMinimum=0.83186  ActiveDisplayYMaximum=1.08242  DataLoggingVariableName=ScopeData13  DataLoggingSaveFormat=Array
  Sum : Sum  Inputs=|+-
  Sum1 : Sum  Inputs=|++
  Voltage : Outport
  wires:
  Sum1/1 -> Product1/2
  Product1/1 -> Scope/1, Voltage/1  "V"
  Sum/1 -> Gain/1
  Low-Pass Filter (Discrete or Continuous)/1 -> Scope1/1, Sum/2
  Constant/1 -> Sum1/2
  Vmeas/1 -> Low-Pass Filter (Discrete or Continuous)/1, Scope2/2
  Gain/1 -> Sum1/1
  Vref/1 -> Sum/1, Product1/1, Scope2/1

== system MicrogridControl/BESS/BESS Integrated3/Detailed/BESS Controller/Grid Forming/Current Limiting/CurrentLimitingMethod/currentLimitAndVirtual/Current Saturation ==
  note: Vs-delV
  Id : Inport
  Iq : Inport  Port=2
  Imaxsat : Inport  Port=3
  Enable : EnablePort
  Compare : Subsystem
  Constant1 : Constant  Value=0
  Constant2 : Constant  Value=0
  If : If
  If Action Subsystem : Subsystem  TreatAsAtomicUnit=on
  If Action Subsystem1 : Subsystem  TreatAsAtomicUnit=on
  Math Function : Math  Operator=hypot
  Merge : Merge
  Merge1 : Merge
  Subtract : Sum  Inputs=+-
  delVd : Outport
  delVq : Outport  Port=2
  idmax : Outport  Port=3
  iqmax : Outport  Port=4
  wires:
  [Imax] -> If Action Subsystem/4(maxI)
  Imaxsat/1 -> Subtract/1, [Imax]
  Merge1/1 -> iqmax/1
  [Isq] -> If Action Subsystem/3(Isq)
  Constant1/1 -> delVd/1
  [Isd] -> If Action Subsystem/2(Isd)
  Merge/1 -> idmax/1
  If Action Subsystem1/2(Iqmax) -> Merge1/2
  Id/1 -> Math Function/1, [Isd]
  [Is] -> If Action Subsystem/1(Is)
  If Action Subsystem/1(Idmax) -> Merge/1
  Compare/1(Out1) -> If/1
  Subtract/1 -> Compare/1(u)
  If Action Subsystem/2(Iqmax) -> Merge1/1
  If/2 -> If Action Subsystem1/Action
  Math Function/1 -> Subtract/2, [Is]
  Constant2/1 -> delVq/1
  If Action Subsystem1/1(Idmax) -> Merge/2
  If/1 -> If Action Subsystem/Action
  Iq/1 -> Math Function/2, [Isq]

== system MicrogridControl/BESS/BESS Integrated3/Detailed/BESS Controller/Grid Forming/Current Limiting/CurrentLimitingMethod/currentLimitAndVirtual/No Fault Ride Through ==
  Id : Inport
  Iq : Inport  Port=2
  Enable : EnablePort
  Constant{1..4} (4 alike) : Constant  Value=0
  Terminator : Terminator
  Terminator1 : Terminator
  delVd : Outport
  delVq : Outport  Port=2
  idmax : Outport  Port=3
  iqmax : Outport  Port=4
  wires:
  Iq/1 -> Terminator1/1
  Id/1 -> Terminator/1
  Constant4/1 -> delVq/1
  Constant1/1 -> delVd/1
  Constant2/1 -> idmax/1
  Constant3/1 -> iqmax/1

== system MicrogridControl/BESS/BESS Integrated3/Detailed/BESS Controller/Grid Forming/Current Limiting/CurrentLimitingMethod/currentLimitAndVirtual/VI ==
  note: X/R ratio
  note: Resistance coefficient
  Id : Inport
  Iq : Inport  Port=2
  Imax : Inport  Port=3
  Enable : EnablePort
  Constant1 : Constant  Value=0
  Constant2 : Constant  Value=0
  Constant3 : Constant  Value=0
  Gain : Gain  Gain=ctLimitVirtualImp
  Gain1 : Gain  Gain=ctLimitXbyR
  Low-Pass Filter : eeGeneralControl/Low-Pass Filter (Discrete or Continuous)  K=1  T=currentVITimeConst  B=inf  A=-inf  init_option=Inherited from block input  x0=0  Ts=-1
  Math Function : Math  Operator=hypot
  Product{,1..3} (4 alike) : Product
  Relay1 : Relay  OnSwitchValue=0.01  OffSwitchValue=-0.1
  Saturation : Saturate  UpperLimit=1  LowerLimit=-1
  Saturation1 : Saturate  UpperLimit=1  LowerLimit=-1
  Sum : Sum  Inputs=|+-
  Sum1 : Sum  Inputs=|+-
  Sum2 : Sum  Inputs=++|
  Switch : Switch  Criteria=u2 > Threshold  SaturateOnIntegerOverflow=off  InputSameDT=off
  delVd : Outport
  delVq : Outport  Port=2
  idmax : Outport  Port=3
  iqmax : Outport  Port=4
  wires:
  Imax/1 -> Sum/2  "IsMaximum"
  Low-Pass Filter/1 -> Sum/1
  Relay1/1 -> Switch/2
  Constant2/1 -> idmax/1
  Constant3/1 -> iqmax/1
  Saturation/1 -> delVd/1
  Constant1/1 -> Switch/3
  Gain/1 -> Switch/1
  Product2/1 -> Sum1/2
  Product1/1 -> Sum2/1
  Saturation1/1 -> delVq/1
  [Igd] -> Product/2, Product1/1
  Switch/1 -> Gain1/1, Product/1, Product3/2
  Math Function/1 -> Low-Pass Filter/1  "Is"
  Iq/1 -> Math Function/2, [Igq]
  [Igq] -> Product2/2, Product3/1
  Product/1 -> Sum1/1
  Sum1/1 -> Saturation/1
  Sum/1 -> Relay1/1, Gain/1
  Sum2/1 -> Saturation1/1
  Id/1 -> [Igd], Math Function/1
  Product3/1 -> Sum2/2
  Gain1/1 -> Product2/1, Product1/2

== system MicrogridControl/BESS/BESS Integrated3/Detailed/BESS Controller/Grid Forming/Current Limiting/CurrentLimitingMethod/currentSaturation/Compare ==
  u : Inport
  AND : Logic  IconShape=distinctive  AllPortsSameDT=off  OutDataTypeStr=boolean
  Compare To Constant : simulink/Logic and Bit Operations/Compare To Constant  relop=>  const=ctLimitDelayTime  OutDataTypeStr=boolean
  Compare To Zero : simulink/Logic and Bit Operations/Compare To Zero  relop=<=  OutDataTypeStr=boolean
  Data Type Conversion : DataTypeConversion  SaturateOnIntegerOverflow=off  RndMeth=Floor
  Data Type Conversion1 : DataTypeConversion  SaturateOnIntegerOverflow=off  RndMeth=Floor
  Discrete-Time Integrator : DiscreteIntegrator  IntegratorMethod=Integration: Backward Euler  ExternalReset=level  SampleTime=currentControlTs  LimitOutput=on  UpperSaturationLimit=ctLimitDelayTime*2  LowerSaturationLimit=0  ICPrevOutput=DiscIntNeverNeededParam  ICPrevScaledInput=DiscIntNeverNeededParam
  Out1 : Outport
  wires:
  Data Type Conversion1/1 -> AND/1, Discrete-Time Integrator/1, Discrete-Time Integrator/2
  Data Type Conversion/1 -> Out1/1
  Discrete-Time Integrator/1 -> Compare To Constant/1
  u/1 -> Compare To Zero/1
  Compare To Constant/1 -> AND/2
  Compare To Zero/1 -> Data Type Conversion1/1
  AND/1 -> Data Type Conversion/1

== system MicrogridControl/BESS/BESS Integrated3/Detailed/BESS Controller/Grid Forming/Current Limiting/CurrentLimitingMethod/currentSaturation/If Action Subsystem ==
  Is : Inport
  Isd : Inport  Port=2
  Isq : Inport  Port=3
  Action Port : ActionPort  ActionPortLabel=if(u1 > 0)
  Constant : Constant  Value=maxSatCurrentLimit
  Divide : Product  Inputs=*/
  Product : Product
  Product1 : Product
  Idmax : Outport
  Iqmax : Outport  Port=2
  wires:
  Product/1 -> Iqmax/1
  Product1/1 -> Idmax/1
  Isq/1 -> Product/2
  Isd/1 -> Product1/1
  Divide/1 -> Product/1, Product1/2
  Is/1 -> Divide/2
  Constant/1 -> Divide/1

== system MicrogridControl/BESS/BESS Integrated3/Detailed/BESS Controller/Grid Forming/Current Limiting/CurrentLimitingMethod/currentSaturation/If Action Subsystem1 ==
  Action Port : ActionPort  ActionPortLabel=else
  Constant3 : Constant  Value=0
  Constant4 : Constant  Value=0
  Idmax : Outport
  Iqmax : Outport  Port=2
  wires:
  Constant3/1 -> Idmax/1
  Constant4/1 -> Iqmax/1

== system MicrogridControl/BESS/BESS Integrated3/Detailed/BESS Controller/Grid Forming/Grid Voltage Reactive Power Support/Modifying Reactive Power Reference/Changing the Power Reference/ActivePowerReference ==
  note: Ensure Pref sign is maintained
  Id : Inport
  Vd : Inport  Port=2
  Pref : Inport  Port=3
  Abs1 : Abs  SaturateOnIntegerOverflow=off
  Abs2 : Abs  SaturateOnIntegerOverflow=off
  Min : MinMax  Inputs=2
  Product : Product
  Product2 : Product
  Saturation : Saturate  UpperLimit=1  LowerLimit=-1
  Sign : Signum
  PrefNew : Outport
  wires:
  Saturation/1 -> PrefNew/1
  Vd/1 -> Product/2
  Abs2/1 -> Min/1
  Product2/1 -> Saturation/1
  Min/1 -> Product2/1
  Product/1 -> Abs2/1
  Abs1/1 -> Min/2
  Sign/1 -> Product2/2
  Id/1 -> Product/1
  Pref/1 -> Sign/1, Abs1/1

== system MicrogridControl/BESS/BESS Integrated3/Detailed/BESS Controller/Grid Forming/Grid Voltage Reactive Power Support/Modifying Reactive Power Reference/Changing the Power Reference/EstimateIdForGivenIq ==
  Iq : Inport
  Add Constant1 : Bias  Bias=1*1  SaturateOnIntegerOverflow=off
  Gain : Gain  Gain=-1
  Gain3 : Gain  Gain=0.9
  Sqrt : Sqrt
  Square : Math  Operator=square
  Id : Outport
  wires:
  Iq/1 -> Square/1
  Add Constant1/1 -> Sqrt/1
  Sqrt/1 -> Gain3/1
  Gain/1 -> Add Constant1/1
  Gain3/1 -> Id/1
  Square/1 -> Gain/1

== system MicrogridControl/BESS/BESS Integrated3/Detailed/BESS Controller/Grid Forming/Grid Voltage Reactive Power Support/Modifying Reactive Power Reference/Changing the Power Reference/EstimateIqForReactivePower ==
  note: Computing minimum reactive power as per GC0137
  Vmin : Inport
  Vd : Inport  Port=2
  Vs : Inport  Port=3
  Abs : Abs  SaturateOnIntegerOverflow=off
  Add : Sum
  Add Constant : Bias  Bias=1  SaturateOnIntegerOverflow=off
  GC0137 line slope : Gain  Gain=-1.4578
  Gain4 : Gain  Gain=1.5
  Saturation : Saturate  UpperLimit=1  LowerLimit=0
  Saturation1 : Saturate  UpperLimit=1  LowerLimit=-1
  Subtract : Sum  Inputs=+-
  Iq : Outport
  wires:
  Add Constant/1 -> Add/2
  Saturation/1 -> Iq/1
  Add/1 -> Saturation/1
  Vd/1 -> Subtract/2
  Vs/1 -> Abs/1
  Vmin/1 -> Subtract/1
  Gain4/1 -> Saturation1/1
  Saturation1/1 -> Add/1
  Subtract/1 -> Gain4/1
  GC0137 line slope/1 -> Add Constant/1
  Abs/1 -> GC0137 line slope/1

== system MicrogridControl/BESS/BESS Integrated3/Detailed/BESS Controller/Grid Forming/Grid Voltage Reactive Power Support/Modifying Reactive Power Reference/Changing the Power Reference/ReactivePowerReference ==
  Vd : Inport
  Iq : Inport  Port=2
  Compute Power : Product
  Constant : Constant  Value=0.3
  Gain2 : Gain  Gain=1.05
  Switch : Switch  Criteria=u2 > Threshold  Threshold=0.3  SaturateOnIntegerOverflow=off  InputSameDT=off
  QrefNew : Outport
  wires:
  Switch/1 -> Compute Power/1
  Vd/1 -> Switch/1, Switch/2
  Iq/1 -> Gain2/1
  Constant/1 -> Switch/3
  Gain2/1 -> Compute Power/2
  Compute Power/1 -> QrefNew/1

== system MicrogridControl/BESS/BESS Integrated3/Detailed/BESS Controller/Grid Forming/Measurement/Frequency Measurement/Frequency Measurement/If Action Subsystem ==
  V : Inport
  Time : Inport  Port=2
  Action Port : ActionPort  ActionPortLabel=if(u1 > 0.9)
  Constant1 : Constant  Value=initialFrequency
  Delay : Delay  DelayLength=1
  Delay1 : Delay  DelayLength=1
  Frequency estimation : Subsystem  TreatAsAtomicUnit=on
  Hit Crossing : HitCross
  Second-Order Filter : eeGeneralControl/Second-Order Filter  Commented=through  FilterType=Low-pass  fn=initialFrequency  Zeta=1  Ts=sampleTime  A0=0  Ph0=0  f0=0  b0=0
  Switch : Switch  Criteria=u2 > Threshold  Threshold=1  SaturateOnIntegerOverflow=off  InputSameDT=off
  Freq : Outport
  wires:
  Switch/1 -> Freq/1
  Constant1/1 -> Switch/3
  Frequency estimation/1(f) -> Switch/1
  Time/1 -> Frequency estimation/3(k), Delay1/1, Switch/2
  V/1 -> Second-Order Filter/1
  Delay/1 -> Frequency estimation/2(sk-1)
  Hit Crossing/1 -> Frequency estimation/Trigger
  Delay1/1 -> Frequency estimation/4(k-1)
  Second-Order Filter/1 -> Hit Crossing/1, Frequency estimation/1(sk), Delay/1

== system MicrogridControl/BESS/BESS Integrated3/Detailed/BESS Controller/Grid Forming/Measurement/Frequency Measurement/Frequency Measurement/If Action Subsystem1 ==
  Action Port : ActionPort  ActionPortLabel=else
  Constant1 : Constant  Value=initialFrequency
  Out1 : Outport
  wires:
  Constant1/1 -> Out1/1
